simulink model "mainmodel"  (R2020a)
settings: Solver=VariableStepAuto  StartTime=0.0  StopTime=10.0  MaxStep=0.01  RelTol=1e-3
PreLoadFcn:
  | theRoadSignal
values from neighbouring files (symbols this model uses):
  b = 40    [theRoadSignal.m]
  k1 = 50    [theRoadSignal.m]
  k2 = 80    [theRoadSignal.m]
  M1 = 100    [theRoadSignal.m]
  M2 = 20    [theRoadSignal.m]
settings Model: Creator=Bhanu  LastModifiedBy=Bhanu
settings DataIOCC: ExternalInput=[t, road]  LoadExternalInput=on

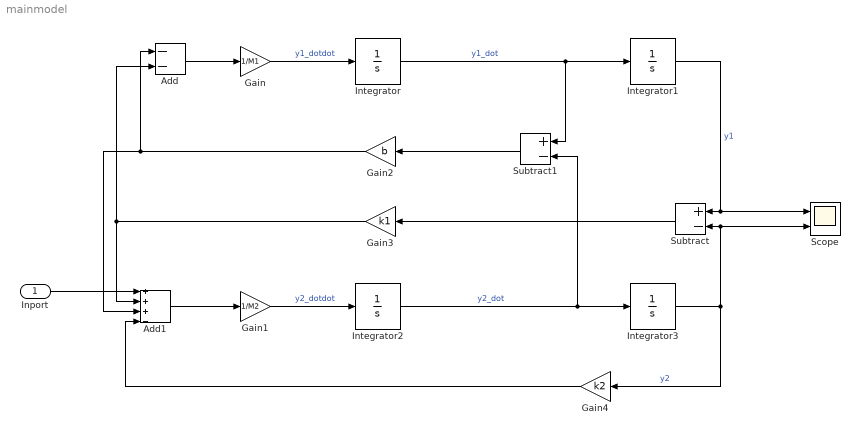
== system mainmodel ==
  Inport : Inport
  Add : Sum  Inputs=--
  Add1 : Sum  Inputs=+++-
  Gain : Gain  Gain=1/M1
  Gain1 : Gain  Gain=1/M2
  Gain2 : Gain  Gain=b
  Gain3 : Gain  Gain=k1
  Gain4 : Gain  Gain=k2
  Integrator{,1..3} (4 alike) : Integrator
  Scope : Scope  NumInputPorts=2
  Subtract : Sum  Inputs=+-
  Subtract1 : Sum  Inputs=+-
  wires:
  Integrator/1 -> Subtract1/1, Integrator1/1  "y1_dot"
  Integrator2/1 -> Subtract1/2, Integrator3/1  "y2_dot"
  Gain1/1 -> Integrator2/1  "y2_dotdot"
  Gain/1 -> Integrator/1  "y1_dotdot"
  Integrator1/1 -> Subtract/1, Scope/1  "y1"
  Integrator3/1 -> Scope/2, Subtract/2, Gain4/1  "y2"
  Add/1 -> Gain/1
  Inport/1 -> Add1/1
  Add1/1 -> Gain1/1
  Subtract1/1 -> Gain2/1
  Gain2/1 -> Add1/3, Add/1
  Subtract/1 -> Gain3/1
  Gain3/1 -> Add1/2, Add/2
  Gain4/1 -> Add1/4
